simulink model "combined_MRAC"  (Simulink 10.3)
settings: Solver=ode45  StartTime=10  StopTime=20  RelTol=1e-3  AbsTol=1e-6
values from neighbouring files (symbols this model uses):
  Af = zeros(nf); Af(1:nf-1, 2:nf) = eye(nf-1); Af(end, :) = -fliplr(den_filtro(2:end))    [combined_MRAC_sim.m]
  alpha = 1    [combined_MRAC_sim.m]
  beta = 1000    [combined_MRAC_sim.m]
  Bf = zeros(nf,1); Bf(end) = 1    [combined_MRAC_sim.m]
  DC = 3    [combined_MRAC_sim.m]
  gamma = 5*eye(2*n)    [combined_MRAC_sim.m]
  kappa = 0.1    [combined_MRAC_sim.m]
  kp = 1/3    (= 0.333333333333)    [combined_MRAC_sim.m]
  l0 = 2    [combined_MRAC_sim.m]
  n = 4    [combined_MRAC_sim.m]
  R0 = 200*eye(2*n)    [combined_MRAC_sim.m]
  sigma = 0.5    [combined_MRAC_sim.m]
  st = 0.01    [combined_MRAC_sim.m]
  tau = 5    [combined_MRAC_sim.m]
  theta0 = zeros(2*n, 1)    [combined_MRAC_sim.m]
libraries: cstblocks x2
settings Model: LogicAnalyzerSignalOrdering=04636dda-aa95-4e8b-bb39-0bd40ee0108f,0649f2ae-a165-4795-88eb-a8023d709948,1767f6c0-72db-4326-990e-1cea0aac2c5e,8ee54cda-48a5-4f61-a93b-b693f9d82bf2,526efd16-2cb2-4f7f-a17b-592242ce68b8,aae53962-6e0f-4536-bb75-dcc56da18767,4b990eb9-e6e9-4be3-a561-dba9f3434993,c301852b-13dd-4bf9-97ec-3918340fcf72,0804b0ab-6626-4093-842a-42967a9eb430,07634013-a215-406c-9446-536cbe8534d0,105c6e3e-79ac-498f-8881-b95e47e9edba,10dc0d5a-646b-48fc-bc01-8c278f0b01d3,284e3033-e2b9-4478-9794-9f1044b479ce,7416a645-b114-49ae-ab40-1077c7b9da29,84f9decd-d03a-4e8c-aff8-17bb0f9b3e63  Creator=Ramon  LastModifiedBy=linco  MultithreadedSim=on
settings SolverCC: AutoScaleAbsTol=off
settings DataIOCC: SaveOutput=off  SaveTime=off
settings OptimizationCC: BlockReduction=off  BooleanDataType=off  InitFltsAndDblsToZero=on
settings DebuggingCC: SaveWithParameterizedLinksMsg=none  SignalResolutionControl=TryResolveAllWithWarning  MultiTaskDSMMsg=warning  MultiTaskCondExecSysMsg=none
settings HardwareCC: TargetUnknown=on
settings RTWCC: TemplateMakefile=grt_vc.tmf

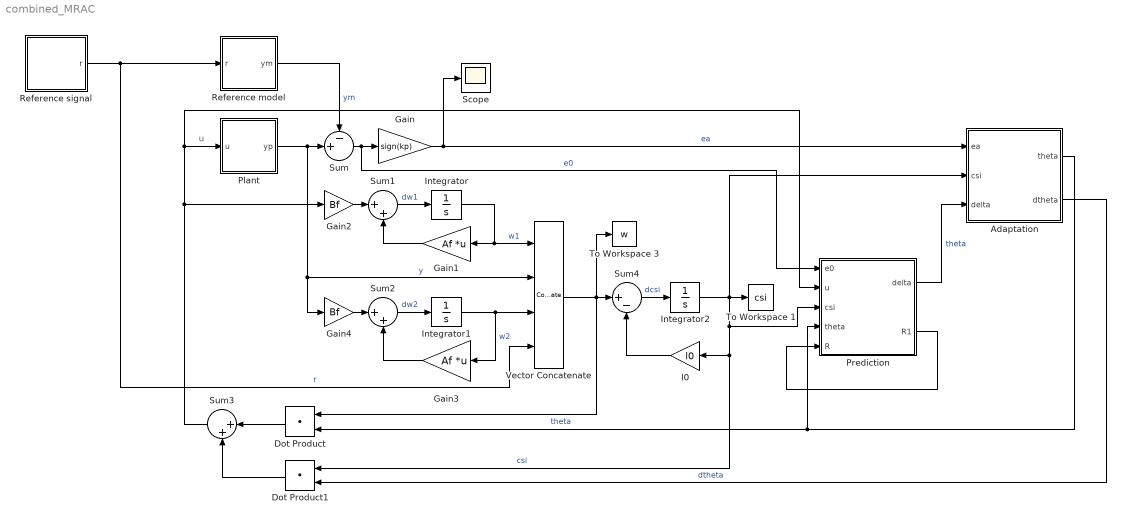
== system combined_MRAC ==
  note: u
  Adaptation : Subsystem
  Dot Product : DotProduct  InputSameDT=on  OutDataTypeStr=Inherit: Inherit via internal rule
  Dot Product1 : DotProduct  InputSameDT=on  OutDataTypeStr=Inherit: Inherit via internal rule
  Gain : Gain  Gain=sign(kp)
  Gain1 : Gain  Gain=Af  Multiplication=Matrix(K*u) (u vector)
  Gain2 : Gain  Gain=Bf
  Gain3 : Gain  Gain=Af  Multiplication=Matrix(K*u) (u vector)
  Gain4 : Gain  Gain=Bf
  Integrator : Integrator
  Integrator1 : Integrator
  Integrator2 : Integrator
  Plant : Subsystem
  Prediction : Subsystem
  Reference model : Subsystem
  Reference signal : Subsystem
  Scope : Scope
  Sum : Sum  Inputs=-+|  InputSameDT=on  SaturateOnIntegerOverflow=on  OutDataTypeStr=Inherit: Same as first input
  Sum1 : Sum  Inputs=|++  InputSameDT=on  SaturateOnIntegerOverflow=on  OutDataTypeStr=Inherit: Same as first input
  Sum2 : Sum  Inputs=|++  InputSameDT=on  SaturateOnIntegerOverflow=on  OutDataTypeStr=Inherit: Same as first input
  Sum3 : Sum  Inputs=|++  InputSameDT=on  SaturateOnIntegerOverflow=on  OutDataTypeStr=Inherit: Same as first input
  Sum4 : Sum  Inputs=|+-  InputSameDT=on  SaturateOnIntegerOverflow=on  OutDataTypeStr=Inherit: Same as first input
  To Workspace 1 : ToWorkspace  VariableName=csi  SampleTime=st
  To Workspace 3 : ToWorkspace  VariableName=w  SampleTime=st
  Vector Concatenate : Concatenate  NumInputs=4
  l0 : Gain  Gain=l0
  wires:
  Reference model/1(ym) -> Sum/1  "ym"
  Plant/1(yp) -> Gain4/1, Vector Concatenate/2, Sum/2  "y"
  Sum3/1 -> Prediction/2(u), Plant/1(u), Gain2/1
  Adaptation/1(theta) -> Dot Product/2, Prediction/4(theta)  "theta"
  Gain/1 -> Adaptation/1(ea), Scope/1  "ea"
  Sum/1 -> Prediction/1(e0), Gain/1  "e0"
  Sum1/1 -> Integrator/1  "dw1"
  Gain2/1 -> Sum1/1
  Integrator/1 -> Vector Concatenate/1, Gain1/1  "w1"
  Gain1/1 -> Sum1/2
  Sum2/1 -> Integrator1/1  "dw2"
  Reference signal/1(r) -> Vector Concatenate/4, Reference model/1(r)  "r"
  Integrator1/1 -> Gain3/1, Vector Concatenate/3  "w2"
  Gain3/1 -> Sum2/2
  Gain4/1 -> Sum2/1
  Vector Concatenate/1 -> Sum4/1, To Workspace 3/1, Dot Product/1
  Integrator2/1 -> Adaptation/2(csi), To Workspace 1/1, Prediction/3(csi), Dot Product1/1, l0/1  "csi"
  Sum4/1 -> Integrator2/1  "dcsi"
  l0/1 -> Sum4/2
  Dot Product/1 -> Sum3/1
  Dot Product1/1 -> Sum3/2
  Adaptation/2(dtheta) -> Dot Product1/2  "dtheta"
  Prediction/1(delta) -> Adaptation/3(delta)  "theta"
  Prediction/2(R1) -> Prediction/5(R)

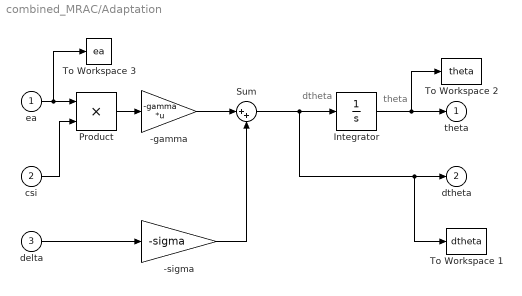
== system combined_MRAC/Adaptation ==
  note: theta
  note: dtheta
  ea : Inport  PortDimensions=1
  csi : Inport  Port=2
  delta : Inport  Port=3
  -gamma : Gain  Gain=-gamma  Multiplication=Matrix(K*u) (u vector)  SaturateOnIntegerOverflow=on  OutDataTypeStr=Inherit: Same as input  ParamDataTypeStr=Inherit: Same as input
  -sigma : Gain  Gain=-sigma  SaturateOnIntegerOverflow=on  OutDataTypeStr=Inherit: Same as input  ParamDataTypeStr=Inherit: Same as input
  Integrator : Integrator  InitialCondition=theta0
  Product : Product  InputSameDT=on  RndMeth=Zero  SaturateOnIntegerOverflow=on  OutDataTypeStr=Inherit: Same as first input
  Sum : Sum  Inputs=|++
  To Workspace 1 : ToWorkspace  VariableName=dtheta  SampleTime=st
  To Workspace 2 : ToWorkspace  VariableName=theta  SampleTime=st
  To Workspace 3 : ToWorkspace  VariableName=ea  SampleTime=st
  theta : Outport  InitialOutput=0  VectorParamsAs1DForOutWhenUnconnected=off
  dtheta : Outport  Port=2  InitialOutput=0  VectorParamsAs1DForOutWhenUnconnected=off
  wires:
  Integrator/1 -> To Workspace 2/1, theta/1
  Sum/1 -> To Workspace 1/1, dtheta/1, Integrator/1
  ea/1 -> Product/1, To Workspace 3/1
  Product/1 -> -gamma/1
  csi/1 -> Product/2
  -gamma/1 -> Sum/1
  delta/1 -> -sigma/1
  -sigma/1 -> Sum/2

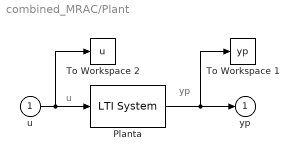
== system combined_MRAC/Plant ==
  note: yp
  note: u
  u : Inport
  Planta : cstblocks/LTI System  sys=P  IC=x0
  To Workspace 1 : ToWorkspace  VariableName=yp  SampleTime=st
  To Workspace 2 : ToWorkspace  VariableName=u  SampleTime=st
  yp : Outport  InitialOutput=0  VectorParamsAs1DForOutWhenUnconnected=off
  wires:
  u/1 -> To Workspace 2/1, Planta/1
  Planta/1 -> yp/1, To Workspace 1/1

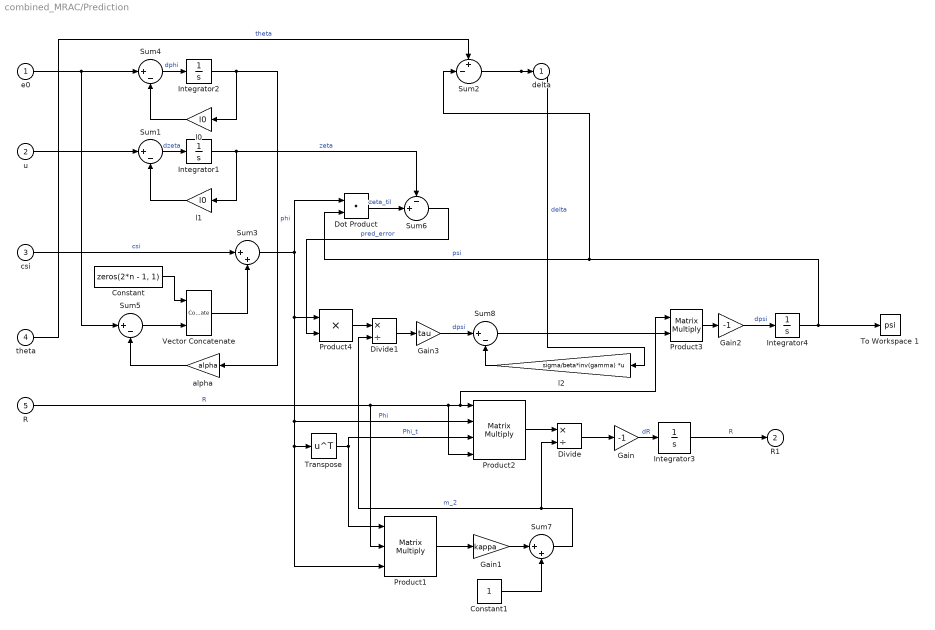
== system combined_MRAC/Prediction ==
  e0 : Inport  PortDimensions=1
  u : Inport  Port=2
  csi : Inport  Port=3
  theta : Inport  Port=4
  R : Inport  Port=5
  Constant : Constant  Value=zeros(2*n - 1, 1)
  Constant1 : Constant
  Divide : Product  Inputs=*/
  Divide1 : Product  Inputs=*/
  Dot Product : DotProduct  InputSameDT=on  OutDataTypeStr=Inherit: Inherit via internal rule
  Gain : Gain  Gain=-1
  Gain1 : Gain  Gain=kappa
  Gain2 : Gain  Gain=-1
  Gain3 : Gain  Gain=tau
  Integrator1 : Integrator
  Integrator2 : Integrator
  Integrator3 : Integrator  InitialCondition=R0
  Integrator4 : Integrator
  Product1 : Product  Inputs=3  Multiplication=Matrix(*)  InputSameDT=on  RndMeth=Zero  SaturateOnIntegerOverflow=on  OutDataTypeStr=Inherit: Same as first input
  Product2 : Product  Inputs=4  Multiplication=Matrix(*)  InputSameDT=on  RndMeth=Zero  SaturateOnIntegerOverflow=on  OutDataTypeStr=Inherit: Same as first input
  Product3 : Product  Multiplication=Matrix(*)  InputSameDT=on  RndMeth=Zero  SaturateOnIntegerOverflow=on  OutDataTypeStr=Inherit: Same as first input
  Product4 : Product  InputSameDT=on  RndMeth=Zero  SaturateOnIntegerOverflow=on  OutDataTypeStr=Inherit: Same as first input
  Sum{1,4..5,8} (4 alike) : Sum  Inputs=|+-  InputSameDT=on  SaturateOnIntegerOverflow=on  OutDataTypeStr=Inherit: Same as first input
  Sum2 : Sum  Inputs=+-|  InputSameDT=on  SaturateOnIntegerOverflow=on  OutDataTypeStr=Inherit: Same as first input
  Sum3 : Sum  Inputs=|++  InputSameDT=on  SaturateOnIntegerOverflow=on  OutDataTypeStr=Inherit: Same as first input
  Sum6 : Sum  Inputs=-+|  InputSameDT=on  SaturateOnIntegerOverflow=on  OutDataTypeStr=Inherit: Same as first input
  Sum7 : Sum  Inputs=|++  InputSameDT=on  SaturateOnIntegerOverflow=on  OutDataTypeStr=Inherit: Same as first input
  To Workspace 1 : ToWorkspace  VariableName=psi  SampleTime=st
  Transpose : Math  Operator=transpose  SaturateOnIntegerOverflow=on
  Vector Concatenate : Concatenate
  alpha : Gain  Gain=alpha
  l0 : Gain  Gain=l0
  l1 : Gain  Gain=l0
  l2 : Gain  Gain=sigma/beta*inv(gamma)  Multiplication=Matrix(K*u) (u vector)
  delta : Outport  InitialOutput=0  VectorParamsAs1DForOutWhenUnconnected=off
  R1 : Outport  Port=2  InitialOutput=0  VectorParamsAs1DForOutWhenUnconnected=off
  wires:
  e0/1 -> Sum5/1, Sum4/1
  Sum4/1 -> Integrator2/1  "dphi"
  l0/1 -> Sum4/2
  Integrator2/1 -> l0/1, alpha/1  "phi"
  l1/1 -> Sum1/2
  u/1 -> Sum1/1
  Sum1/1 -> Integrator1/1  "dzeta"
  Integrator1/1 -> Sum6/1, l1/1  "zeta"
  Product2/1 -> Divide/1
  Gain/1 -> Integrator3/1  "dR"
  theta/1 -> Sum2/1  "theta"
  Sum2/1 -> l2/1, delta/1  "delta"
  csi/1 -> Sum3/1  "csi"
  Dot Product/1 -> Sum6/2  "zeta_til"
  Constant/1 -> Vector Concatenate/1
  Vector Concatenate/1 -> Sum3/2
  Sum3/1 -> Product2/2, Transpose/1, Product1/3, Product4/1, Dot Product/1  "Phi"
  Sum5/1 -> Vector Concatenate/2
  alpha/1 -> Sum5/2
  Sum6/1 -> Product4/2  "pred_error"
  Divide/1 -> Gain/1
  Product1/1 -> Gain1/1
  Gain1/1 -> Sum7/1
  Constant1/1 -> Sum7/2
  Sum7/1 -> Divide1/2, Divide/2  "m_2"
  Transpose/1 -> Product1/1, Product2/3  "Phi_t"
  Integrator4/1 -> To Workspace 1/1, Dot Product/2, Sum2/2  "psi"
  Product3/1 -> Gain2/1
  Gain2/1 -> Integrator4/1  "dpsi"
  Gain3/1 -> Sum8/1  "dpsi"
  Sum8/1 -> Product3/2
  Product4/1 -> Divide1/1
  Divide1/1 -> Gain3/1
  l2/1 -> Sum8/2
  Integrator3/1 -> R1/1  "R"
  R/1 -> Product3/1, Product2/1, Product2/4, Product1/2  "R"

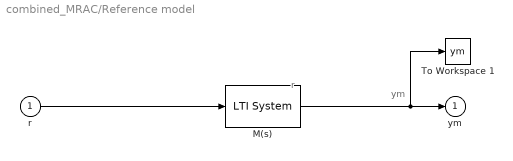
== system combined_MRAC/Reference model ==
  note: r
  note: ym
  r : Inport
  M(s) : cstblocks/LTI System  sys=M  IC=xm0
  To Workspace 1 : ToWorkspace  VariableName=ym  SampleTime=st
  ym : Outport  InitialOutput=0  VectorParamsAs1DForOutWhenUnconnected=off
  wires:
  M(s)/1 -> To Workspace 1/1, ym/1
  r/1 -> M(s)/1

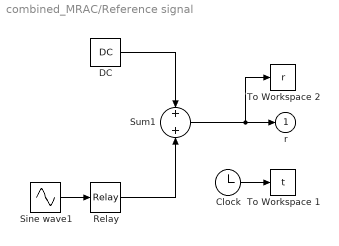
== system combined_MRAC/Reference signal ==
  Clock : Clock
  DC : Constant  Value=DC
  Relay : Relay  OnOutputValue=10  OffOutputValue=-10
  Sine wave1 : Sin  Frequency=0.1*pi  SampleTime=0
  Sum1 : Sum  InputSameDT=on  SaturateOnIntegerOverflow=on  OutDataTypeStr=Inherit: Same as first input
  To Workspace 1 : ToWorkspace  VariableName=t  SampleTime=st
  To Workspace 2 : ToWorkspace  VariableName=r  SampleTime=st
  r : Outport  InitialOutput=0  VectorParamsAs1DForOutWhenUnconnected=off
  wires:
  DC/1 -> Sum1/1
  Sum1/1 -> r/1, To Workspace 2/1
  Clock/1 -> To Workspace 1/1
  Relay/1 -> Sum1/2
  Sine wave1/1 -> Relay/1
